simulink model "TransmCtrl_V1"  (R2018a)
settings: Solver=VariableStepAuto  StartTime=0.0  StopTime=10.0  FixedStep=sampletime  RelTol=1e-3  EnableMultiTasking=on
PreLoadFcn:
  | TransmCtrl_V1_PreLoad
values from neighbouring files (symbols this model uses):
  downtab = [0 5 20 35 ... (first row only)    [TransmCtrl_V1_PreLoad.m]
  downth = [0; 5; 40; 50; 90; 100]    [TransmCtrl_V1_PreLoad.m]
  uptab = [10 30 50 1.0E+6 ... (first row only)    [TransmCtrl_V1_PreLoad.m]
  upth = [0; 25; 35; 50; 90; 100]    [TransmCtrl_V1_PreLoad.m]
libraries: simulink x2
settings Model: Creator=IAEC nishito  LastModifiedBy=nishito
settings DataIOCC: LimitDataPoints=on  SaveFormat=Array  SignalLoggingSaveFormat=ModelDataLogs  SaveOutput=off  SaveTime=off
settings OptimizationCC: DefaultParameterBehavior=Inlined  ExpressionDepthLimit=2147483647  LifeSpan=inf
settings DebuggingCC: UnderspecifiedInitializationDetection=Classic  MergeDetectMultiDrivingBlocksExec=none  SolverPrmCheckMsg=warning  FcnCallInpInsideContextMsg=warning  StateNameClashWarn=warning  SFUnexpectedBacktrackingDiag=warning  SFNoUnconditionalDefaultTransitionDiag=warning  SFExecutionAtInitializationDiag=none
settings HardwareCC: ProdBitPerPointer=32  ProdBitPerSizeT=32  ProdBitPerPtrDiffT=32  ProdLargestAtomicFloat=None  ProdIntDivRoundTo=Undefined  ProdEndianess=Unspecified  ProdWordSize=32  ProdHWDeviceType=32-bit Generic
settings ModelReferenceCC: UpdateModelReferenceTargets=IfOutOfDate  PropagateSignalLabelsOutOfModel=off
settings CodeAppCC: StateflowObjectComments=on
settings GRTTargetCC: TargetLangStandard=C89/C90 (ANSI)  GeneratePreprocessorConditionals=Disable all  CombineOutputUpdateFcns=off  GRTInterface=on
settings ConfigComp: CovMetricSettings=dw  CovHtmlReporting=on  CovSaveCumulativeToWorkspaceVar=on  CovSaveSingleToWorkspaceVar=on  CovExternalEMLEnable=off

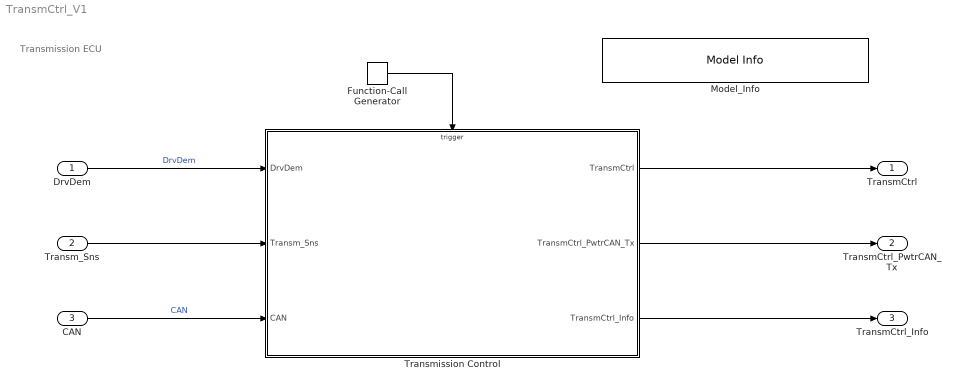
== system TransmCtrl_V1 ==
  note: Transmission ECU
  DrvDem : Inport  OutDataTypeStr=Bus: Driver_demand_Bus
      settings: AttributesFormatString=%<OutDataTypeStr>
  Transm_Sns : Inport  Port=2  OutDataTypeStr=Bus: Transm_sensor_Bus
      settings: AttributesFormatString=%<OutDataTypeStr>
  CAN : Inport  Port=3  OutDataTypeStr=Bus: CAN_Bus
      settings: AttributesFormatString=<%<OutDataTypeStr>>
  Function-Call Generator : simulink/Ports & Subsystems/Function-Call Generator  sample_time=0.01  numberOfIterations=1
      settings: AttributesFormatString=<sample_time=%<sample_time>>
  Model_Info : simulink/Model-Wide Utilities/Model Info  Frame=on  DisplayStringWithTags=|  HorizontalTextAlignment=Left  LeftAlignmentValue=0.02
      | Version  %<ModelVersion>
      | LastModifided by %<LastModifiedBy>  Date %<LastModificationDate>
      | Description  %<Description>
  Transmission Control : Subsystem
  TransmCtrl : Outport  OutDataTypeStr=Bus: TransmCtrl_Bus
      settings: AttributesFormatString=<%<OutDataTypeStr>>
  TransmCtrl_PwtrCAN_Tx : Outport  Port=2  OutDataTypeStr=Bus: TransmCtrl_PwtrCAN_Tx_Bus
      settings: AttributesFormatString=<%<OutDataTypeStr>>
  TransmCtrl_Info : Outport  Port=3  OutDataTypeStr=Bus: TransmCtrl_Info_Bus
      settings: AttributesFormatString=<%<OutDataTypeStr>>
  wires:
  CAN/1 -> Transmission Control/3(CAN)  "CAN"
  DrvDem/1 -> Transmission Control/1(DrvDem)  "DrvDem"
  Transm_Sns/1 -> Transmission Control/2(Transm_Sns)
  Function-Call Generator/1 -> Transmission Control/Trigger
  Transmission Control/2(TransmCtrl_PwtrCAN_Tx) -> TransmCtrl_PwtrCAN_Tx/1
  Transmission Control/1(TransmCtrl) -> TransmCtrl/1
  Transmission Control/3(TransmCtrl_Info) -> TransmCtrl_Info/1

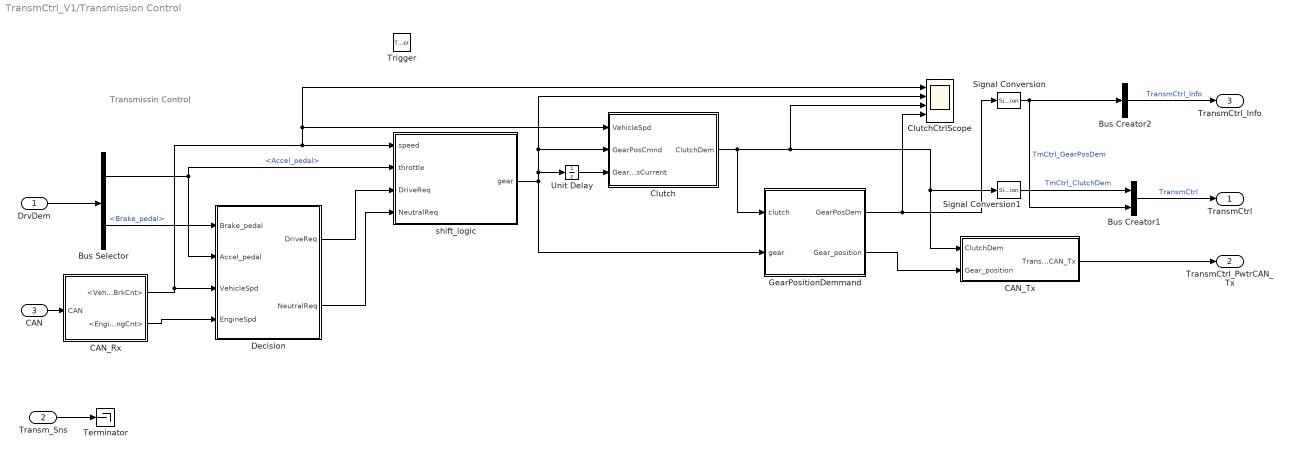
== system TransmCtrl_V1/Transmission Control ==
  note: Transmissin Control
  DrvDem : Inport
  Transm_Sns : Inport  Port=2
  CAN : Inport  Port=3
  Trigger : TriggerPort  TriggerType=function-call  VariantControl=Variant  PortDimensions=1
  Bus Creator1 : BusCreator  Inputs=2  OutDataTypeStr=Bus: TransmCtrl_Bus
      settings: AttributesFormatString=%<OutDataTypeStr>
  Bus Creator2 : BusCreator  Inputs=1  OutDataTypeStr=Bus: TransmCtrl_Info_Bus
      settings: AttributesFormatString=%<OutDataTypeStr>
  Bus Selector : BusSelector  OutputSignals=Accel_pedal,Brake_pedal
  CAN_Rx : Subsystem
  CAN_Tx : Subsystem
  Clutch : Subsystem
  ClutchCtrlScope : Scope  NumInputPorts=4
  Decision : Subsystem
  GearPositionDemmand : Subsystem
  Signal Conversion : SignalConversion  OverrideOpt=off
  Signal Conversion1 : SignalConversion  OverrideOpt=off
  Terminator : Terminator
  Unit Delay : UnitDelay  SampleTime=-1
  shift_logic : Stateflow chart  TreatAsAtomicUnit=on
      settings: AttributesFormatString=%<SystemSampleTime>
  TransmCtrl : Outport
  TransmCtrl_PwtrCAN_Tx : Outport  Port=2
  TransmCtrl_Info : Outport  Port=3
  wires:
  DrvDem/1 -> Bus Selector/1
  Transm_Sns/1 -> Terminator/1
  Unit Delay/1 -> Clutch/3(GearPosCurrent)
  shift_logic/1(gear) -> GearPositionDemmand/2(gear), ClutchCtrlScope/2, Clutch/2(GearPosCmnd), Unit Delay/1
  Clutch/1(ClutchDem) -> GearPositionDemmand/1(clutch), ClutchCtrlScope/3, CAN_Tx/1(ClutchDem), Signal Conversion1/1
  Decision/2(NeutralReq) -> shift_logic/4(NeutralReq)
  GearPositionDemmand/1(GearPosDem) -> ClutchCtrlScope/4, Signal Conversion/1
  Bus Selector/1 -> shift_logic/2(throttle), Decision/2(Accel_pedal)  "<Accel_pedal>"
  Decision/1(DriveReq) -> shift_logic/3(DriveReq)
  Bus Selector/2 -> Decision/1(Brake_pedal)  "<Brake_pedal>"
  Bus Creator1/1 -> TransmCtrl/1  "TransmCtrl"
  Bus Creator2/1 -> TransmCtrl_Info/1  "TransmCtrl_Info"
  GearPositionDemmand/2(Gear_position) -> CAN_Tx/2(Gear_position)
  CAN_Tx/1(TransmCtrl_PwtrCAN_Tx) -> TransmCtrl_PwtrCAN_Tx/1
  CAN_Rx/1(<Vehicle_speed_BrkCnt>) -> Clutch/1(VehicleSpd), ClutchCtrlScope/1, shift_logic/1(speed), Decision/3(VehicleSpd)
  CAN/1 -> CAN_Rx/1(CAN)
  CAN_Rx/2(<Engine_speed_EngCnt>) -> Decision/4(EngineSpd)
  Signal Conversion/1 -> Bus Creator1/2, Bus Creator2/1  "TmCtrl_GearPosDem"
  Signal Conversion1/1 -> Bus Creator1/1  "TmCtrl_ClutchDem"

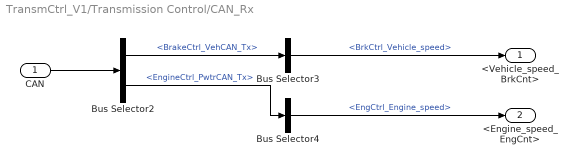
== system TransmCtrl_V1/Transmission Control/CAN_Rx ==
  CAN : Inport
  Bus Selector2 : BusSelector  OutputSignals=VehCAN.BrakeCtrl_VehCAN_Tx,PwtrCAN.EngineCtrl_PwtrCAN_Tx
  Bus Selector3 : BusSelector  OutputSignals=BrkCtrl_Vehicle_speed
  Bus Selector4 : BusSelector  OutputSignals=EngCtrl_Engine_speed
  <Vehicle_speed_BrkCnt> : Outport
  <Engine_speed_EngCnt> : Outport  Port=2
  wires:
  Bus Selector3/1 -> <Vehicle_speed_BrkCnt>/1  "<BrkCtrl_Vehicle_speed>"
  CAN/1 -> Bus Selector2/1
  Bus Selector2/1 -> Bus Selector3/1  "<BrakeCtrl_VehCAN_Tx>"
  Bus Selector2/2 -> Bus Selector4/1  "<EngineCtrl_PwtrCAN_Tx>"
  Bus Selector4/1 -> <Engine_speed_EngCnt>/1  "<EngCtrl_Engine_speed>"

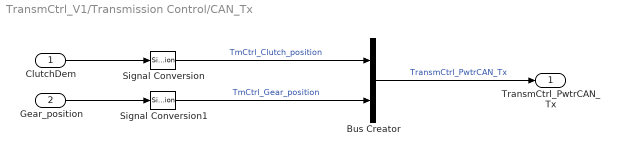
== system TransmCtrl_V1/Transmission Control/CAN_Tx ==
  ClutchDem : Inport
  Gear_position : Inport  Port=2
  Bus Creator : BusCreator  Inputs=2  OutDataTypeStr=Bus: TransmCtrl_PwtrCAN_Tx_Bus
      settings: AttributesFormatString=%<OutDataTypeStr>
  Signal Conversion : SignalConversion  OverrideOpt=off
  Signal Conversion1 : SignalConversion  OverrideOpt=off
  TransmCtrl_PwtrCAN_Tx : Outport
  wires:
  Bus Creator/1 -> TransmCtrl_PwtrCAN_Tx/1  "TransmCtrl_PwtrCAN_Tx"
  ClutchDem/1 -> Signal Conversion/1
  Gear_position/1 -> Signal Conversion1/1
  Signal Conversion/1 -> Bus Creator/1  "TmCtrl_Clutch_position"
  Signal Conversion1/1 -> Bus Creator/2  "TmCtrl_Gear_position"

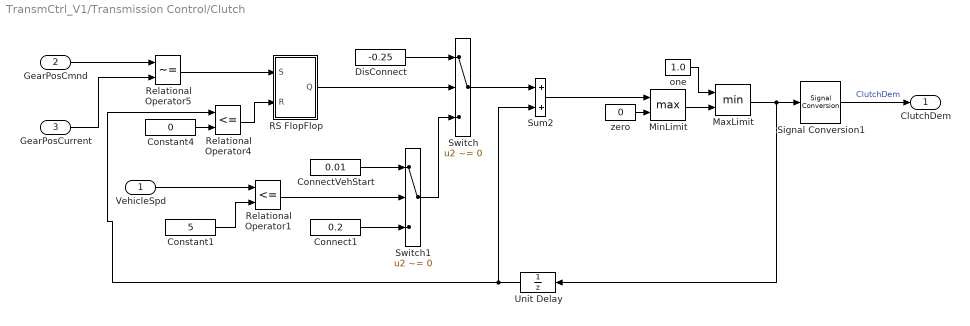
== system TransmCtrl_V1/Transmission Control/Clutch ==
  VehicleSpd : Inport
  GearPosCmnd : Inport  Port=2
  GearPosCurrent : Inport  Port=3
  Connect1 : Constant  Value=0.2
  ConnectVehStart : Constant  Value=0.01
  Constant1 : Constant  Value=5
  Constant4 : Constant  Value=0
  DisConnect : Constant  Value=-0.25
  MaxLimit : MinMax  Inputs=2
  MinLimit : MinMax  Function=max  Inputs=2
  RS FlopFlop : Subsystem
  Relational Operator1 : RelationalOperator  Operator=<=  OutDataTypeStr=boolean  RndMeth=Nearest
  Relational Operator4 : RelationalOperator  Operator=<=  OutDataTypeStr=boolean  RndMeth=Nearest
  Relational Operator5 : RelationalOperator  Operator=~=  OutDataTypeStr=boolean  RndMeth=Nearest
  Signal Conversion1 : SignalConversion  OverrideOpt=off
  Sum2 : Sum
  Switch : Switch  Criteria=u2 ~= 0  Threshold=0.5  SaturateOnIntegerOverflow=on
      settings: AttributesFormatString=<%<Criteria>>
  Switch1 : Switch  Criteria=u2 ~= 0  Threshold=0.5  SaturateOnIntegerOverflow=on
      settings: AttributesFormatString=<%<Criteria>>
  Unit Delay : UnitDelay  InitialCondition=1  SampleTime=-1
  one : Constant  Value=1.0
  zero : Constant  Value=0
  ClutchDem : Outport
  wires:
  GearPosCurrent/1 -> Relational Operator5/2
  Relational Operator5/1 -> RS FlopFlop/1(S)
  GearPosCmnd/1 -> Relational Operator5/1
  DisConnect/1 -> Switch/1
  Signal Conversion1/1 -> ClutchDem/1  "ClutchDem"
  RS FlopFlop/1(Q) -> Switch/2
  ConnectVehStart/1 -> Switch1/1
  Switch/1 -> Sum2/1
  Sum2/1 -> MinLimit/1
  Unit Delay/1 -> Sum2/2, Relational Operator4/1
  Constant4/1 -> Relational Operator4/2
  MaxLimit/1 -> Unit Delay/1, Signal Conversion1/1
  Relational Operator4/1 -> RS FlopFlop/2(R)
  MinLimit/1 -> MaxLimit/2
  zero/1 -> MinLimit/2
  one/1 -> MaxLimit/1
  VehicleSpd/1 -> Relational Operator1/1
  Constant1/1 -> Relational Operator1/2
  Relational Operator1/1 -> Switch1/2
  Switch1/1 -> Switch/3
  Connect1/1 -> Switch1/3

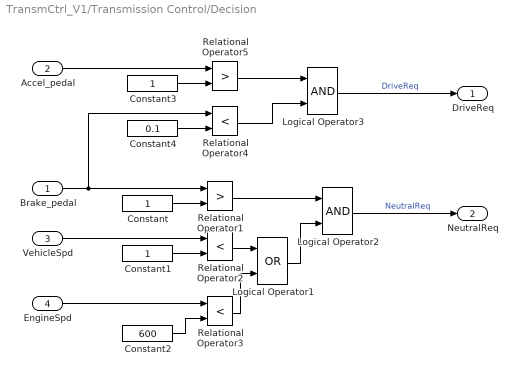
== system TransmCtrl_V1/Transmission Control/Decision ==
  Brake_pedal : Inport
  Accel_pedal : Inport  Port=2
  VehicleSpd : Inport  Port=3
  EngineSpd : Inport  Port=4
  Constant : Constant
  Constant1 : Constant
  Constant2 : Constant  Value=600
  Constant3 : Constant
  Constant4 : Constant  Value=0.1
  Logical Operator1 : Logic  Operator=OR  AllPortsSameDT=off  OutDataTypeStr=boolean
  Logical Operator2 : Logic  AllPortsSameDT=off  OutDataTypeStr=boolean
  Logical Operator3 : Logic  AllPortsSameDT=off  OutDataTypeStr=boolean
  Relational Operator1 : RelationalOperator  Operator=>  OutDataTypeStr=boolean  RndMeth=Nearest
  Relational Operator2 : RelationalOperator  Operator=<  OutDataTypeStr=boolean  RndMeth=Nearest
  Relational Operator3 : RelationalOperator  Operator=<  OutDataTypeStr=boolean  RndMeth=Nearest
  Relational Operator4 : RelationalOperator  Operator=<  OutDataTypeStr=boolean  RndMeth=Nearest
  Relational Operator5 : RelationalOperator  Operator=>  OutDataTypeStr=boolean  RndMeth=Nearest
  DriveReq : Outport
  NeutralReq : Outport  Port=2
  wires:
  Constant2/1 -> Relational Operator3/2
  Logical Operator1/1 -> Logical Operator2/2
  Constant3/1 -> Relational Operator5/2
  EngineSpd/1 -> Relational Operator3/1
  Constant/1 -> Relational Operator1/2
  Relational Operator1/1 -> Logical Operator2/1
  Logical Operator2/1 -> NeutralReq/1  "NeutralReq"
  Relational Operator3/1 -> Logical Operator1/2
  Constant1/1 -> Relational Operator2/2
  Brake_pedal/1 -> Relational Operator4/1, Relational Operator1/1
  Relational Operator2/1 -> Logical Operator1/1
  Logical Operator3/1 -> DriveReq/1  "DriveReq"
  VehicleSpd/1 -> Relational Operator2/1
  Accel_pedal/1 -> Relational Operator5/1
  Constant4/1 -> Relational Operator4/2
  Relational Operator5/1 -> Logical Operator3/1
  Relational Operator4/1 -> Logical Operator3/2

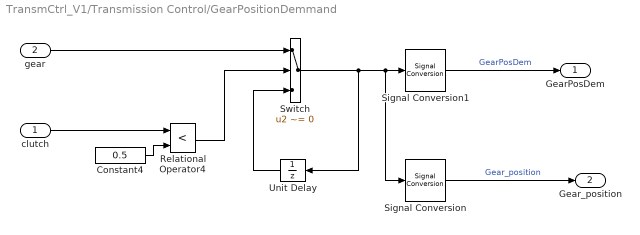
== system TransmCtrl_V1/Transmission Control/GearPositionDemmand ==
  clutch : Inport
  gear : Inport  Port=2
  Constant4 : Constant  Value=0.5
  Relational Operator4 : RelationalOperator  Operator=<  OutDataTypeStr=boolean  RndMeth=Nearest
  Signal Conversion : SignalConversion  OverrideOpt=off
  Signal Conversion1 : SignalConversion  OverrideOpt=off
  Switch : Switch  Criteria=u2 ~= 0  Threshold=0.5  SaturateOnIntegerOverflow=on
      settings: AttributesFormatString=<%<Criteria>>
  Unit Delay : UnitDelay  SampleTime=-1
  GearPosDem : Outport
  Gear_position : Outport  Port=2
  wires:
  Signal Conversion/1 -> Gear_position/1  "Gear_position"
  Signal Conversion1/1 -> GearPosDem/1  "GearPosDem"
  gear/1 -> Switch/1
  clutch/1 -> Relational Operator4/1
  Switch/1 -> Signal Conversion/1, Signal Conversion1/1, Unit Delay/1
  Constant4/1 -> Relational Operator4/2
  Relational Operator4/1 -> Switch/2
  Unit Delay/1 -> Switch/3

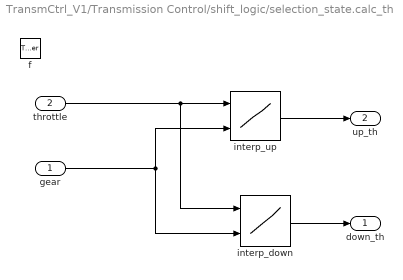
== system TransmCtrl_V1/Transmission Control/shift_logic/selection_state.calc_th ==
  gear : Inport
  throttle : Inport  Port=2
  f : TriggerPort  TriggerType=function-call  VariantControl=Variant
      settings: CopyFcn=Stateflow.SLINSF.SimulinkMan.removeBlockPreDeleteFcn  PreDeleteFcn=Stateflow.SLINSF.SimulinkMan.unsafePredeleteFcn
  interp_down : Lookup_n-D  BreakpointsForDimension1=downth  BreakpointsForDimension2=[1:4]  Table=downtab  InputSameDT=on
  interp_up : Lookup_n-D  BreakpointsForDimension1=upth  BreakpointsForDimension2=[1:4]  Table=uptab  InputSameDT=on
  down_th : Outport
  up_th : Outport  Port=2
  wires:
  gear/1 -> interp_up/2, interp_down/2
  throttle/1 -> interp_up/1, interp_down/1
  interp_down/1 -> down_th/1
  interp_up/1 -> up_th/1

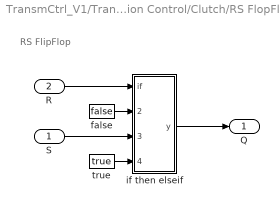
== system TransmCtrl_V1/Transmission Control/Clutch/RS FlopFlop ==
  note: RS FlipFlop
  S : Inport
  R : Inport  Port=2
  false : Constant  Value=false
  if then elseif : Subsystem  mask(if then elseif){}
  true : Constant  Value=true
  Q : Outport
  wires:
  S/1 -> if then elseif/3(elseif)
  R/1 -> if then elseif/1(if)
  if then elseif/1(y) -> Q/1
  false/1 -> if then elseif/2(then1)
  true/1 -> if then elseif/4(then2)

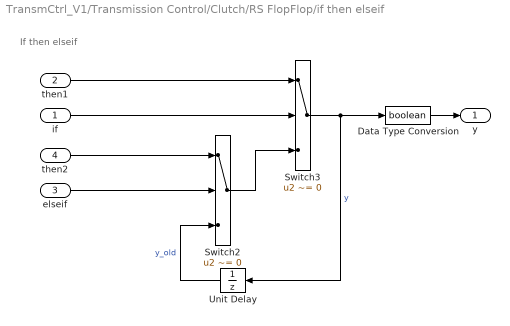
== system TransmCtrl_V1/Transmission Control/Clutch/RS FlopFlop/if then elseif ==
  note: If then elseif
  if : Inport
  then1 : Inport  Port=2
  elseif : Inport  Port=3
  then2 : Inport  Port=4
  Data Type Conversion : DataTypeConversion  OutDataTypeStr=boolean
  Switch2 : Switch  Criteria=u2 ~= 0  Threshold=0.5  SaturateOnIntegerOverflow=on
      settings: AttributesFormatString=<%<Criteria>>
  Switch3 : Switch  Criteria=u2 ~= 0  Threshold=0.5  SaturateOnIntegerOverflow=on
      settings: AttributesFormatString=<%<Criteria>>
  Unit Delay : UnitDelay  SampleTime=-1
      settings: AttributesFormatString=<initial=%<X0>>\n<tsample=%<SampleTime>>
  y : Outport
  wires:
  Data Type Conversion/1 -> y/1
  Switch2/1 -> Switch3/3
  if/1 -> Switch3/2
  Unit Delay/1 -> Switch2/3  "y_old"
  Switch3/1 -> Data Type Conversion/1, Unit Delay/1  "y"
  then1/1 -> Switch3/1
  elseif/1 -> Switch2/2
  then2/1 -> Switch2/1

== stateflow chart TransmCtrl_V1/Transmission Control/shift_logic ==
  settings: sampleTime=0.04
  state gear_state [parallel]
    settings: executionOrder=1
    state neutral
      en:
      gear=0;
    state fourth
      entry: gear = 4;
    state third
      entry: gear = 3;
    state second
      entry: gear = 2;
    state first
      entry: gear = 1;
    (default) -> neutral
    first -> neutral [order 2] : [NeutralReq]
    neutral -> first : [DriveReq]
    second -> third [order 1] : UP
    first -> second [order 1] : UP
    third -> fourth [order 1] : UP
    third -> second [order 2] : DOWN
    fourth -> third : DOWN
    second -> first [order 2] : DOWN
  state selection_state [parallel]
    during: [down_th,up_th] = calc_th(gear,throttle);
    settings: executionOrder=2
    state steady_state
    state upshifting
    state downshifting
    state [down_th,up_th] = calc_th(gear,throttle) [function]
    (default) -> steady_state
    steady_state -> upshifting [order 1] : [(speed > up_th)&&(speed > 5)]
    steady_state -> downshifting [order 2] : [speed < down_th]
    downshifting -> steady_state [order 2] : [speed > down_th]
    downshifting -> steady_state [order 1] : after(TWAIT,tick)
        | [speed <= down_th]
        | {gear_state.DOWN;}
    upshifting -> steady_state [order 1] : after(TWAIT,tick)
        | [speed >= up_th]
        | {gear_state.UP;}
    upshifting -> steady_state [order 2] : [speed < up_th]
  data: gear function_input; throttle function_input; down_th function_output; up_th function_output; speed input double; gear output double [1..4]; TWAIT parameter uint8; up_th local double; down_th local double; throttle input; DriveReq input; NeutralReq input
  events: DOWN local EITHER_EDGE_EVENT; UP local EITHER_EDGE_EVENT
